simulink model "Comparison_to_Nest_Synapse"  (R2020b)
settings: Solver=FixedStepAuto  StartTime=0.0  StopTime=0.4  FixedStep=0.0001  RelTol=1e-3
undefined symbols (not defined in the file or in its folder): heaviside
libraries: NeuroModelerLibrary x9, simulink x3
settings Model: Creator=Александра  LastModifiedBy=Александра

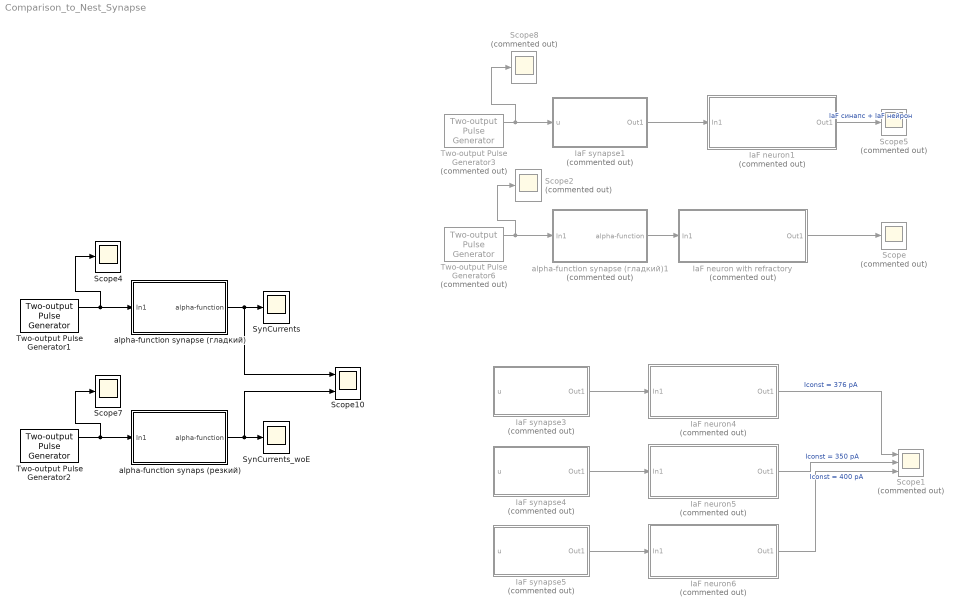
== system Comparison_to_Nest_Synapse ==
  IaF neuron with refractory : Subsystem  Commented=on  mask{tau_m=0.01, Cm=250e-12, I_const=376e-12, E_L=-0.070, V_reset=-0.070, V_th=-0.055, tau_ref=0.002}
      mask prompts: tau_m "Membrane time constatnt"; Cm "Membrane capacity"; I_const "Constant input current"; E_L "Resting membrane potential"; V_reset "Reset membrane potential"; V_th "Threshold potential"; tau_ref "Refractory period"
  IaF neuron1 : Subsystem  Commented=on  mask{tau_m=0.01, Cm=250e-12, I_const=0, E_L=-0.070, V_reset=-0.10, V_th=-0.055}
      mask prompts: tau_m "Membrane time constatnt"; Cm "Membrane capacity"; I_const "Constant input current"; E_L "Resting membrane potential"; V_reset "Reset membrane potential"; V_th "Threshold potential"
  IaF neuron4 : Subsystem  Commented=on  mask{tau_m=0.010, Cm=250e-12, I_const=376e-12, E_L=-0.070, V_reset=-0.070, V_th=-0.055}
      mask prompts: tau_m "Membrane time constatnt"; Cm "Membrane capacity"; I_const "Constant input current"; E_L "Resting membrane potential"; V_reset "Reset membrane potential"; V_th "Threshold potential"
  IaF neuron5 : Subsystem  Commented=on  mask{tau_m=0.010, Cm=250e-12, I_const=350e-12, E_L=-0.070, V_reset=-0.070, V_th=-0.055}
      mask prompts: tau_m "Membrane time constatnt"; Cm "Membrane capacity"; I_const "Constant input current"; E_L "Resting membrane potential"; V_reset "Reset membrane potential"; V_th "Threshold potential"
  IaF neuron6 : Subsystem  Commented=on  mask{tau_m=0.010, Cm=250e-12, I_const=400e-12, E_L=-0.070, V_reset=-0.070, V_th=-0.055}
      mask prompts: tau_m "Membrane time constatnt"; Cm "Membrane capacity"; I_const "Constant input current"; E_L "Resting membrane potential"; V_reset "Reset membrane potential"; V_th "Threshold potential"
  IaF synapse1 : Subsystem  Commented=on  mask{tau_syn=2e-3, I_syn=1, weight=1, delay=1e-3}
      mask prompts: tau_syn "Rise time of the excitatory synaptic alpha function"; I_syn "Synaptic current amplitude"
  IaF synapse3 : Subsystem  Commented=on  mask{tau_syn=2e-3, I_syn=1e-8, weight=1, delay=1e-3}
      mask prompts: tau_syn "Rise time of the excitatory synaptic alpha function"; I_syn "Synaptic current amplitude"
  IaF synapse4 : Subsystem  Commented=on  mask{tau_syn=2e-3, I_syn=1e-8, weight=1, delay=1e-3}
      mask prompts: tau_syn "Rise time of the excitatory synaptic alpha function"; I_syn "Synaptic current amplitude"
  IaF synapse5 : Subsystem  Commented=on  mask{tau_syn=2e-3, I_syn=1e-8, weight=1, delay=1e-3}
      mask prompts: tau_syn "Rise time of the excitatory synaptic alpha function"; I_syn "Synaptic current amplitude"
  Scope{,2,5,8} (4 alike) : Scope  Commented=on
  Scope1 : Scope  Commented=on  NumInputPorts=3
  Scope10 : Scope  NumInputPorts=2
  Scope4 : Scope
  Scope7 : Scope
  SynCurrents : Scope
  SynCurrents_woE : Scope
  Two-output Pulse Generator1 : NeuroModelerLibrary/Support/Two-output Pulse Generator  A=1  P1=200  P2=200  PW=1  ST=0.001  OOn1=0.1  OOff1=1.0  OOn2=0.1  OOff2=0.2
  Two-output Pulse Generator2 : NeuroModelerLibrary/Support/Two-output Pulse Generator  A=1  P1=200  P2=200  PW=1  ST=0.001  OOn1=0.1  OOff1=1.0  OOn2=0.1  OOff2=0.2
  Two-output Pulse Generator3 : NeuroModelerLibrary/Support/Two-output Pulse Generator  Commented=on  A=1  P1=200  P2=200  PW=1  ST=0.001  OOn1=0.1  OOff1=1.0  OOn2=0.1  OOff2=0.2
  Two-output Pulse Generator6 : NeuroModelerLibrary/Support/Two-output Pulse Generator  Commented=on  A=1  P1=200  P2=200  PW=1  ST=0.001  OOn1=0.1  OOff1=1.0  OOn2=0.1  OOff2=0.2
  alpha-function synaps (резкий) : Subsystem
  alpha-function synapse (гладкий) : Subsystem
  alpha-function synapse (гладкий)1 : Subsystem  Commented=on
  wires:
  alpha-function synapse (гладкий)1/1(alpha-function) -> IaF neuron with refractory/1(In1)
  IaF neuron4/1(Out1) -> Scope1/1  "Iconst = 376 pA"
  IaF synapse3/1(Out1) -> IaF neuron4/1(In1)
  IaF synapse4/1(Out1) -> IaF neuron5/1(In1)
  IaF synapse5/1(Out1) -> IaF neuron6/1(In1)
  IaF neuron5/1(Out1) -> Scope1/2  "Iconst = 350 pA"
  IaF neuron6/1(Out1) -> Scope1/3  "Iconst = 400 pA"
  alpha-function synapse (гладкий)/1(alpha-function) -> Scope10/1, SynCurrents/1
  Two-output Pulse Generator1/1 -> Scope4/1, alpha-function synapse (гладкий)/1(In1)
  Two-output Pulse Generator2/1 -> Scope7/1, alpha-function synaps (резкий)/1(In1)
  alpha-function synaps (резкий)/1(alpha-function) -> Scope10/2, SynCurrents_woE/1
  Two-output Pulse Generator6/1 -> alpha-function synapse (гладкий)1/1(In1), Scope2/1
  IaF neuron1/1(Out1) -> Scope5/1  "IaF синапс + IaF нейрон"
  IaF synapse1/1(Out1) -> IaF neuron1/1(In1)
  Two-output Pulse Generator3/1 -> Scope8/1, IaF synapse1/1(u)
  IaF neuron with refractory/1(Out1) -> Scope/1

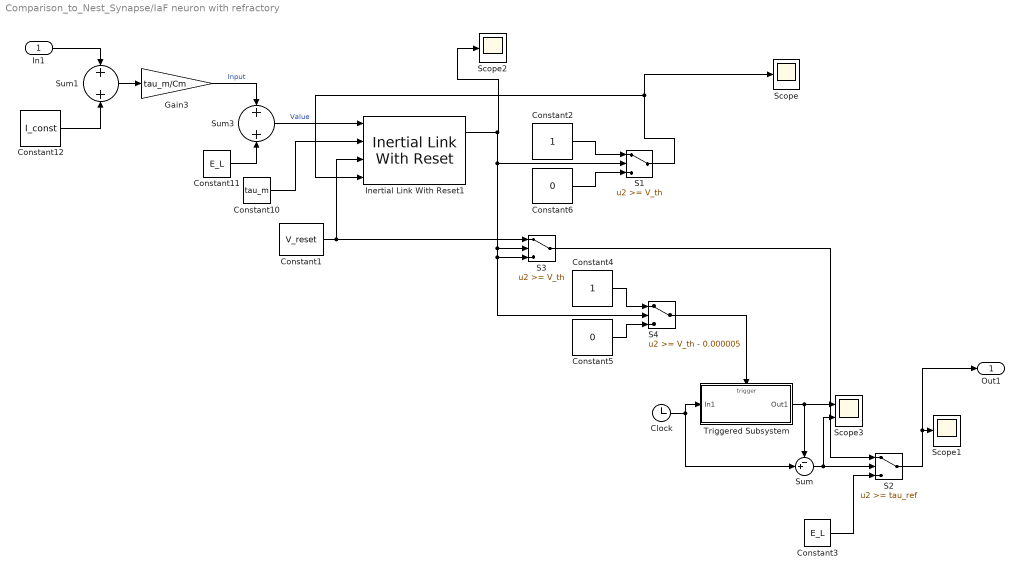
== system Comparison_to_Nest_Synapse/IaF neuron with refractory ==
  In1 : Inport
  Clock : Clock
  Constant1 : Constant  Value=V_reset
  Constant10 : Constant  Value=tau_m
  Constant11 : Constant  Value=E_L
  Constant12 : Constant  Value=I_const
  Constant2 : Constant
  Constant3 : Constant  Value=E_L
  Constant4 : Constant
  Constant5 : Constant  Value=0
  Constant6 : Constant  Value=0
  Gain3 : Gain  Gain=tau_m/Cm
  Inertial Link With Reset1 : NeuroModelerLibrary/Support/Inertial Link With Reset  SystemSampleTime=-1  VariantActivationTime=update diagram  Latency=0  AutoFrameSizeCalculation=off
  S1 : Switch  Threshold=V_th  SaturateOnIntegerOverflow=on  InputSameDT=on
  S2 : Switch  Threshold=tau_ref  SaturateOnIntegerOverflow=on  InputSameDT=on
  S3 : Switch  Threshold=V_th  SaturateOnIntegerOverflow=on  InputSameDT=on
  S4 : Switch  Threshold=V_th - 0.000005  SaturateOnIntegerOverflow=on  InputSameDT=on
  Scope : Scope
  Scope1 : Scope
  Scope2 : Scope
  Scope3 : Scope  NumInputPorts=2
  Sum : Sum  Inputs=-+|
  Sum1 : Sum
  Sum3 : Sum
  Triggered Subsystem : Subsystem  TreatAsAtomicUnit=on
  Out1 : Outport
  wires:
  Constant11/1 -> Sum3/2
  Constant10/1 -> Inertial Link With Reset1/2
  In1/1 -> Sum1/1
  Sum1/1 -> Gain3/1
  Constant12/1 -> Sum1/2
  Constant2/1 -> S1/1
  Constant6/1 -> S1/3
  Sum3/1 -> Inertial Link With Reset1/1  "Value"
  Constant1/1 -> S3/1, Inertial Link With Reset1/3
  S1/1 -> Inertial Link With Reset1/4, Scope/1
  S3/1 -> S2/1
  Gain3/1 -> Sum3/1  "Input"
  Triggered Subsystem/1(Out1) -> Scope3/1, Sum/1
  Clock/1 -> Sum/2, Triggered Subsystem/1(In1)
  Sum/1 -> Scope3/2, S2/2
  S2/1 -> Out1/1, Scope1/1
  Constant3/1 -> S2/3
  Constant4/1 -> S4/1
  Inertial Link With Reset1/1 -> Scope2/1, S4/2, S3/3, S3/2, S1/2
  Constant5/1 -> S4/3
  S4/1 -> Triggered Subsystem/Trigger

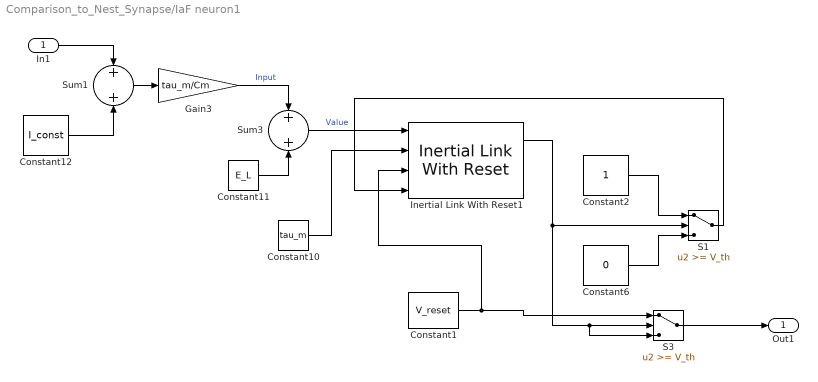
== system Comparison_to_Nest_Synapse/IaF neuron1 ==
  In1 : Inport
  Constant1 : Constant  Value=V_reset
  Constant10 : Constant  Value=tau_m
  Constant11 : Constant  Value=E_L
  Constant12 : Constant  Value=I_const
  Constant2 : Constant
  Constant6 : Constant  Value=0
  Gain3 : Gain  Gain=tau_m/Cm
  Inertial Link With Reset1 : NeuroModelerLibrary/Support/Inertial Link With Reset  SystemSampleTime=-1  VariantActivationTime=update diagram  Latency=0  AutoFrameSizeCalculation=off
  S1 : Switch  Threshold=V_th  SaturateOnIntegerOverflow=on  InputSameDT=on
  S3 : Switch  Threshold=V_th  SaturateOnIntegerOverflow=on  InputSameDT=on
  Sum1 : Sum
  Sum3 : Sum
  Out1 : Outport
  wires:
  Constant11/1 -> Sum3/2
  Constant10/1 -> Inertial Link With Reset1/2
  In1/1 -> Sum1/1
  Sum1/1 -> Gain3/1
  Constant12/1 -> Sum1/2
  Constant2/1 -> S1/1
  Constant6/1 -> S1/3
  Sum3/1 -> Inertial Link With Reset1/1  "Value"
  Inertial Link With Reset1/1 -> S1/2, S3/3, S3/2
  Constant1/1 -> Inertial Link With Reset1/3, S3/1
  S1/1 -> Inertial Link With Reset1/4
  S3/1 -> Out1/1
  Gain3/1 -> Sum3/1  "Input"

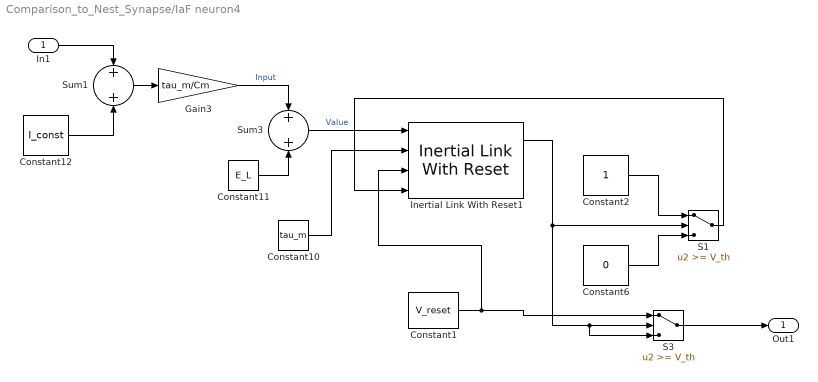
== system Comparison_to_Nest_Synapse/IaF neuron4 ==
  In1 : Inport
  Constant1 : Constant  Value=V_reset
  Constant10 : Constant  Value=tau_m
  Constant11 : Constant  Value=E_L
  Constant12 : Constant  Value=I_const
  Constant2 : Constant
  Constant6 : Constant  Value=0
  Gain3 : Gain  Gain=tau_m/Cm
  Inertial Link With Reset1 : NeuroModelerLibrary/Support/Inertial Link With Reset  SystemSampleTime=-1  VariantActivationTime=update diagram  Latency=0  AutoFrameSizeCalculation=off
  S1 : Switch  Threshold=V_th  SaturateOnIntegerOverflow=on  InputSameDT=on
  S3 : Switch  Threshold=V_th  SaturateOnIntegerOverflow=on  InputSameDT=on
  Sum1 : Sum
  Sum3 : Sum
  Out1 : Outport
  wires:
  Constant11/1 -> Sum3/2
  Constant10/1 -> Inertial Link With Reset1/2
  In1/1 -> Sum1/1
  Sum1/1 -> Gain3/1
  Constant12/1 -> Sum1/2
  Constant2/1 -> S1/1
  Constant6/1 -> S1/3
  Sum3/1 -> Inertial Link With Reset1/1  "Value"
  Inertial Link With Reset1/1 -> S1/2, S3/3, S3/2
  Constant1/1 -> Inertial Link With Reset1/3, S3/1
  S1/1 -> Inertial Link With Reset1/4
  S3/1 -> Out1/1
  Gain3/1 -> Sum3/1  "Input"

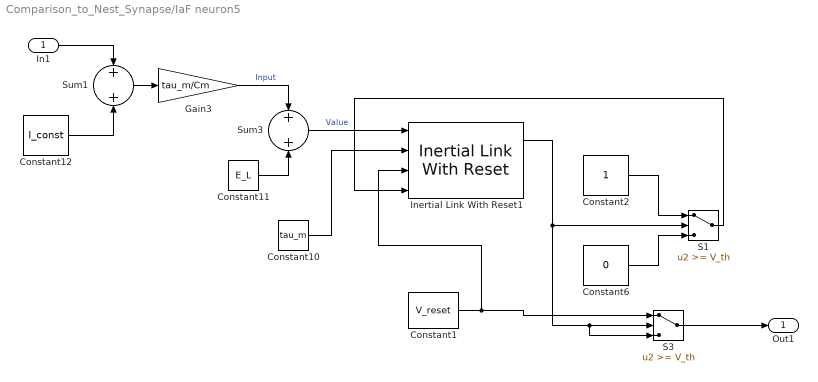
== system Comparison_to_Nest_Synapse/IaF neuron5 ==
  In1 : Inport
  Constant1 : Constant  Value=V_reset
  Constant10 : Constant  Value=tau_m
  Constant11 : Constant  Value=E_L
  Constant12 : Constant  Value=I_const
  Constant2 : Constant
  Constant6 : Constant  Value=0
  Gain3 : Gain  Gain=tau_m/Cm
  Inertial Link With Reset1 : NeuroModelerLibrary/Support/Inertial Link With Reset  SystemSampleTime=-1  VariantActivationTime=update diagram  Latency=0  AutoFrameSizeCalculation=off
  S1 : Switch  Threshold=V_th  SaturateOnIntegerOverflow=on  InputSameDT=on
  S3 : Switch  Threshold=V_th  SaturateOnIntegerOverflow=on  InputSameDT=on
  Sum1 : Sum
  Sum3 : Sum
  Out1 : Outport
  wires:
  Constant11/1 -> Sum3/2
  Constant10/1 -> Inertial Link With Reset1/2
  In1/1 -> Sum1/1
  Sum1/1 -> Gain3/1
  Constant12/1 -> Sum1/2
  Constant2/1 -> S1/1
  Constant6/1 -> S1/3
  Sum3/1 -> Inertial Link With Reset1/1  "Value"
  Inertial Link With Reset1/1 -> S1/2, S3/3, S3/2
  Constant1/1 -> Inertial Link With Reset1/3, S3/1
  S1/1 -> Inertial Link With Reset1/4
  S3/1 -> Out1/1
  Gain3/1 -> Sum3/1  "Input"

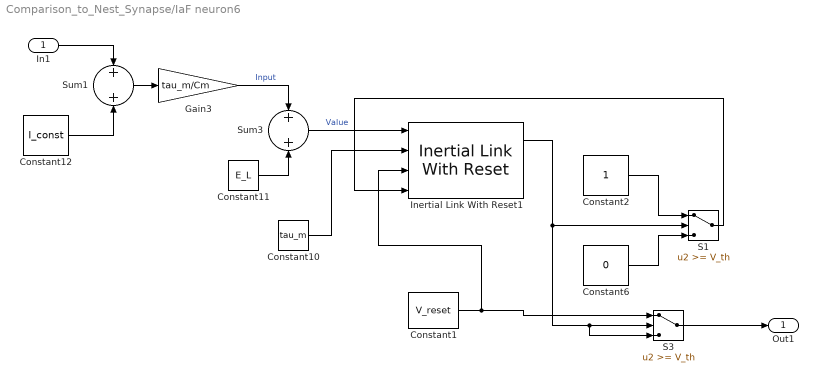
== system Comparison_to_Nest_Synapse/IaF neuron6 ==
  In1 : Inport
  Constant1 : Constant  Value=V_reset
  Constant10 : Constant  Value=tau_m
  Constant11 : Constant  Value=E_L
  Constant12 : Constant  Value=I_const
  Constant2 : Constant
  Constant6 : Constant  Value=0
  Gain3 : Gain  Gain=tau_m/Cm
  Inertial Link With Reset1 : NeuroModelerLibrary/Support/Inertial Link With Reset  SystemSampleTime=-1  VariantActivationTime=update diagram  Latency=0  AutoFrameSizeCalculation=off
  S1 : Switch  Threshold=V_th  SaturateOnIntegerOverflow=on  InputSameDT=on
  S3 : Switch  Threshold=V_th  SaturateOnIntegerOverflow=on  InputSameDT=on
  Sum1 : Sum
  Sum3 : Sum
  Out1 : Outport
  wires:
  Constant11/1 -> Sum3/2
  Constant10/1 -> Inertial Link With Reset1/2
  In1/1 -> Sum1/1
  Sum1/1 -> Gain3/1
  Constant12/1 -> Sum1/2
  Constant2/1 -> S1/1
  Constant6/1 -> S1/3
  Sum3/1 -> Inertial Link With Reset1/1  "Value"
  Inertial Link With Reset1/1 -> S1/2, S3/3, S3/2
  Constant1/1 -> Inertial Link With Reset1/3, S3/1
  S1/1 -> Inertial Link With Reset1/4
  S3/1 -> Out1/1
  Gain3/1 -> Sum3/1  "Input"

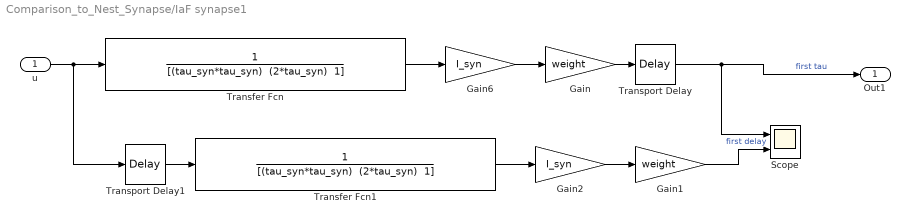
== system Comparison_to_Nest_Synapse/IaF synapse1 ==
  u : Inport
  Gain : Gain  Gain=weight
  Gain1 : Gain  Gain=weight
  Gain2 : Gain  Gain=I_syn
  Gain6 : Gain  Gain=I_syn
  Scope : Scope  NumInputPorts=2
  Transfer Fcn : TransferFcn  Denominator="[(tau_syn*tau_syn)  (2*tau_syn)  1]"
  Transfer Fcn1 : TransferFcn  Denominator="[(tau_syn*tau_syn)  (2*tau_syn)  1]"
  Transport Delay : TransportDelay  DelayTime=delay
  Transport Delay1 : TransportDelay  DelayTime=delay
  Out1 : Outport
  wires:
  Transport Delay/1 -> Scope/1, Out1/1  "first tau"
  Gain/1 -> Transport Delay/1
  Gain6/1 -> Gain/1
  Transfer Fcn/1 -> Gain6/1
  u/1 -> Transport Delay1/1, Transfer Fcn/1
  Transfer Fcn1/1 -> Gain2/1
  Gain2/1 -> Gain1/1
  Transport Delay1/1 -> Transfer Fcn1/1
  Gain1/1 -> Scope/2  "first delay"

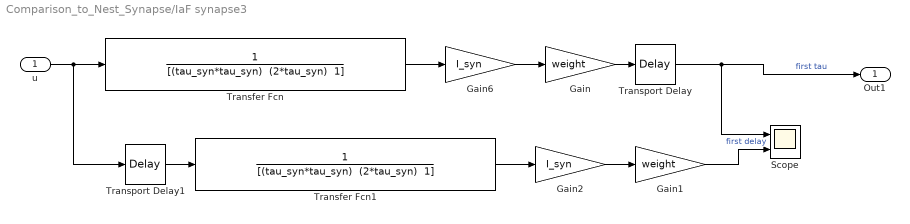
== system Comparison_to_Nest_Synapse/IaF synapse3 ==
  u : Inport
  Gain : Gain  Gain=weight
  Gain1 : Gain  Gain=weight
  Gain2 : Gain  Gain=I_syn
  Gain6 : Gain  Gain=I_syn
  Scope : Scope  NumInputPorts=2
  Transfer Fcn : TransferFcn  Denominator="[(tau_syn*tau_syn)  (2*tau_syn)  1]"
  Transfer Fcn1 : TransferFcn  Denominator="[(tau_syn*tau_syn)  (2*tau_syn)  1]"
  Transport Delay : TransportDelay  DelayTime=delay
  Transport Delay1 : TransportDelay  DelayTime=delay
  Out1 : Outport
  wires:
  Transport Delay/1 -> Scope/1, Out1/1  "first tau"
  Gain/1 -> Transport Delay/1
  Gain6/1 -> Gain/1
  Transfer Fcn/1 -> Gain6/1
  u/1 -> Transport Delay1/1, Transfer Fcn/1
  Transfer Fcn1/1 -> Gain2/1
  Gain2/1 -> Gain1/1
  Transport Delay1/1 -> Transfer Fcn1/1
  Gain1/1 -> Scope/2  "first delay"

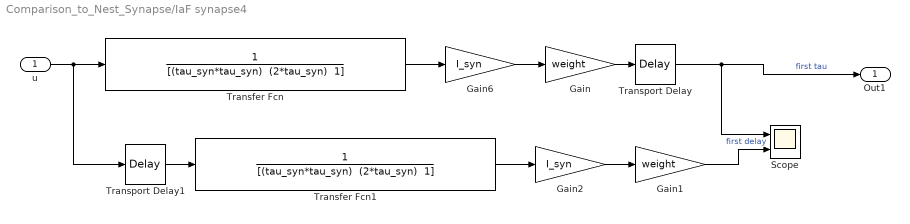
== system Comparison_to_Nest_Synapse/IaF synapse4 ==
  u : Inport
  Gain : Gain  Gain=weight
  Gain1 : Gain  Gain=weight
  Gain2 : Gain  Gain=I_syn
  Gain6 : Gain  Gain=I_syn
  Scope : Scope  NumInputPorts=2
  Transfer Fcn : TransferFcn  Denominator="[(tau_syn*tau_syn)  (2*tau_syn)  1]"
  Transfer Fcn1 : TransferFcn  Denominator="[(tau_syn*tau_syn)  (2*tau_syn)  1]"
  Transport Delay : TransportDelay  DelayTime=delay
  Transport Delay1 : TransportDelay  DelayTime=delay
  Out1 : Outport
  wires:
  Transport Delay/1 -> Scope/1, Out1/1  "first tau"
  Gain/1 -> Transport Delay/1
  Gain6/1 -> Gain/1
  Transfer Fcn/1 -> Gain6/1
  u/1 -> Transport Delay1/1, Transfer Fcn/1
  Transfer Fcn1/1 -> Gain2/1
  Gain2/1 -> Gain1/1
  Transport Delay1/1 -> Transfer Fcn1/1
  Gain1/1 -> Scope/2  "first delay"

== system Comparison_to_Nest_Synapse/IaF synapse5 ==
  u : Inport
  Gain : Gain  Gain=weight
  Gain1 : Gain  Gain=weight
  Gain2 : Gain  Gain=I_syn
  Gain6 : Gain  Gain=I_syn
  Scope : Scope  NumInputPorts=2
  Transfer Fcn : TransferFcn  Denominator="[(tau_syn*tau_syn)  (2*tau_syn)  1]"
  Transfer Fcn1 : TransferFcn  Denominator="[(tau_syn*tau_syn)  (2*tau_syn)  1]"
  Transport Delay : TransportDelay  DelayTime=delay
  Transport Delay1 : TransportDelay  DelayTime=delay
  Out1 : Outport
  wires:
  Transport Delay/1 -> Scope/1, Out1/1  "first tau"
  Gain/1 -> Transport Delay/1
  Gain6/1 -> Gain/1
  Transfer Fcn/1 -> Gain6/1
  u/1 -> Transport Delay1/1, Transfer Fcn/1
  Transfer Fcn1/1 -> Gain2/1
  Gain2/1 -> Gain1/1
  Transport Delay1/1 -> Transfer Fcn1/1
  Gain1/1 -> Scope/2  "first delay"

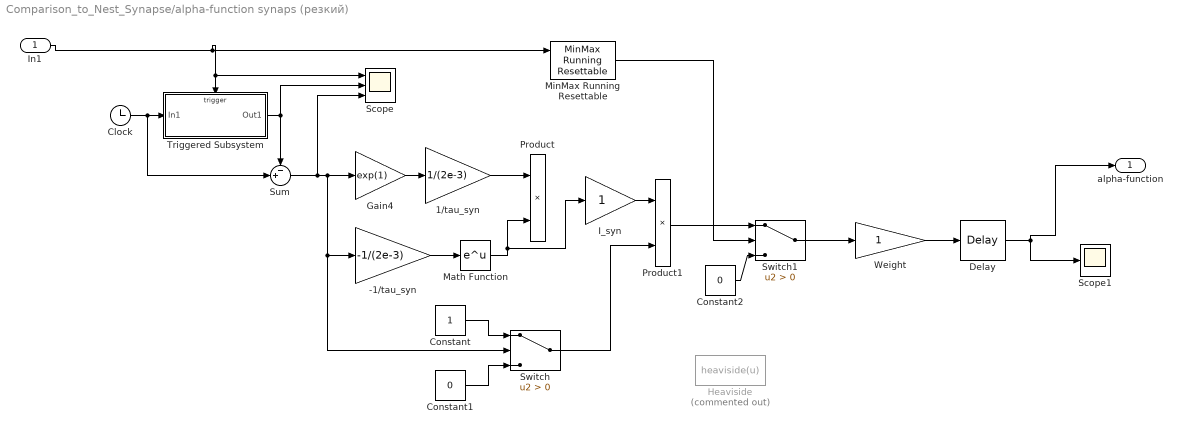
== system Comparison_to_Nest_Synapse/alpha-function synaps (резкий) ==
  In1 : Inport
  -1/tau_syn : Gain  Gain=-1/(2e-3)
  1/tau_syn : Gain  Gain=1/(2e-3)
  Clock : Clock
  Constant : Constant
  Constant1 : Constant  Value=0
  Constant2 : Constant  Value=0
  Delay : TransportDelay  DelayTime=0.001
  Gain4 : Gain  Gain=exp(1)
  Heaviside : MATLABFcn  Commented=on  MATLABFcn=heaviside(u)  OutputSignalType=real  Output1D=off
  I_syn : Gain
  Math Function : Math  SaturateOnIntegerOverflow=on
  MinMax Running Resettable : simulink/Math Operations/MinMax Running Resettable  Function=max  vinit=0.0
  Product : Product
  Product1 : Product
  Scope : Scope  NumInputPorts=3
  Scope1 : Scope
  Sum : Sum  Inputs=-+|
  Switch : Switch  Criteria=u2 > Threshold
  Switch1 : Switch  Criteria=u2 > Threshold
  Triggered Subsystem : Subsystem  TreatAsAtomicUnit=on
  Weight : Gain
  alpha-function : Outport
  wires:
  I_syn/1 -> Product1/1
  1/tau_syn/1 -> Product/1
  Weight/1 -> Delay/1
  Sum/1 -> Scope/3, Switch/2, -1/tau_syn/1, Gain4/1
  Gain4/1 -> 1/tau_syn/1
  -1/tau_syn/1 -> Math Function/1
  Math Function/1 -> I_syn/1, Product/2
  Switch/1 -> Product1/2
  Clock/1 -> Sum/2, Triggered Subsystem/1(In1)
  In1/1 -> Scope/1, Triggered Subsystem/Trigger, MinMax Running Resettable/1
  Triggered Subsystem/1(Out1) -> Sum/1, Scope/2
  Constant1/1 -> Switch/3
  Constant/1 -> Switch/1
  Constant2/1 -> Switch1/3
  Product1/1 -> Switch1/1
  MinMax Running Resettable/1 -> Switch1/2
  Switch1/1 -> Weight/1
  Delay/1 -> alpha-function/1, Scope1/1

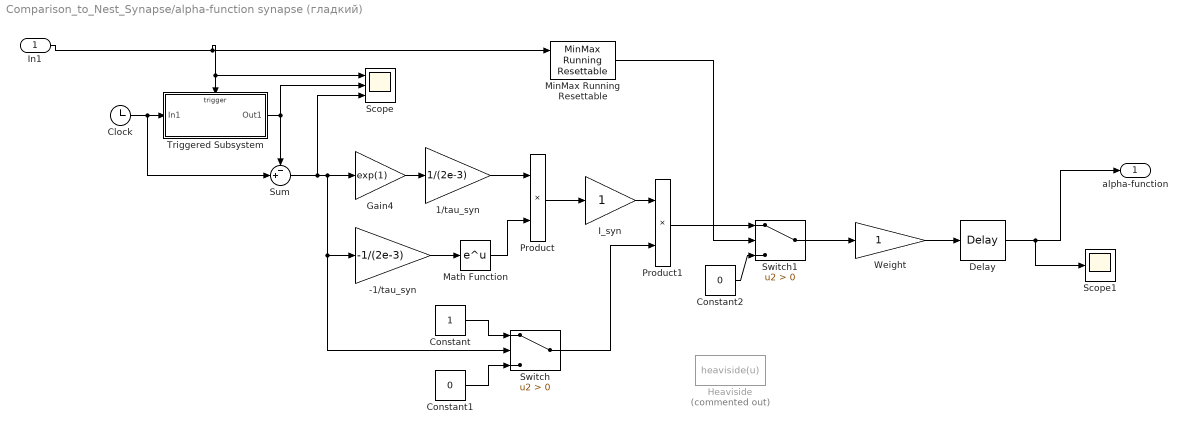
== system Comparison_to_Nest_Synapse/alpha-function synapse (гладкий) ==
  In1 : Inport
  -1/tau_syn : Gain  Gain=-1/(2e-3)
  1/tau_syn : Gain  Gain=1/(2e-3)
  Clock : Clock
  Constant : Constant
  Constant1 : Constant  Value=0
  Constant2 : Constant  Value=0
  Delay : TransportDelay  DelayTime=0.001
  Gain4 : Gain  Gain=exp(1)
  Heaviside : MATLABFcn  Commented=on  MATLABFcn=heaviside(u)  OutputSignalType=real  Output1D=off
  I_syn : Gain
  Math Function : Math  SaturateOnIntegerOverflow=on
  MinMax Running Resettable : simulink/Math Operations/MinMax Running Resettable  Function=max  vinit=0.0
  Product : Product
  Product1 : Product
  Scope : Scope  NumInputPorts=3
  Scope1 : Scope
  Sum : Sum  Inputs=-+|
  Switch : Switch  Criteria=u2 > Threshold
  Switch1 : Switch  Criteria=u2 > Threshold
  Triggered Subsystem : Subsystem  TreatAsAtomicUnit=on
  Weight : Gain
  alpha-function : Outport
  wires:
  I_syn/1 -> Product1/1
  1/tau_syn/1 -> Product/1
  Weight/1 -> Delay/1
  Sum/1 -> Scope/3, Switch/2, -1/tau_syn/1, Gain4/1
  Gain4/1 -> 1/tau_syn/1
  -1/tau_syn/1 -> Math Function/1
  Math Function/1 -> Product/2
  Switch/1 -> Product1/2
  Clock/1 -> Sum/2, Triggered Subsystem/1(In1)
  In1/1 -> Scope/1, Triggered Subsystem/Trigger, MinMax Running Resettable/1
  Triggered Subsystem/1(Out1) -> Sum/1, Scope/2
  Constant1/1 -> Switch/3
  Constant/1 -> Switch/1
  Product/1 -> I_syn/1
  Constant2/1 -> Switch1/3
  Product1/1 -> Switch1/1
  MinMax Running Resettable/1 -> Switch1/2
  Switch1/1 -> Weight/1
  Delay/1 -> Scope1/1, alpha-function/1

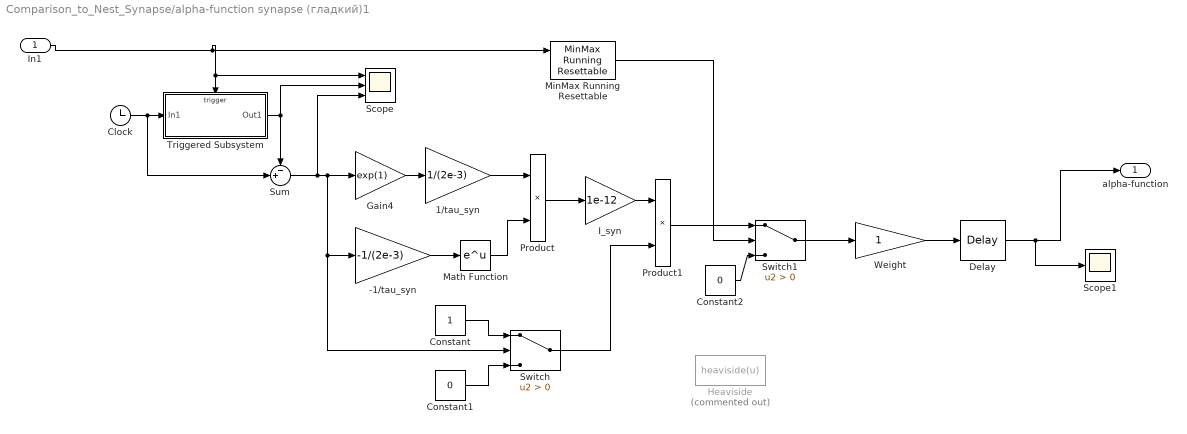
== system Comparison_to_Nest_Synapse/alpha-function synapse (гладкий)1 ==
  In1 : Inport
  -1/tau_syn : Gain  Gain=-1/(2e-3)
  1/tau_syn : Gain  Gain=1/(2e-3)
  Clock : Clock
  Constant : Constant
  Constant1 : Constant  Value=0
  Constant2 : Constant  Value=0
  Delay : TransportDelay  DelayTime=0.001
  Gain4 : Gain  Gain=exp(1)
  Heaviside : MATLABFcn  Commented=on  MATLABFcn=heaviside(u)  OutputSignalType=real  Output1D=off
  I_syn : Gain  Gain=1e-12
  Math Function : Math  SaturateOnIntegerOverflow=on
  MinMax Running Resettable : simulink/Math Operations/MinMax Running Resettable  Function=max  vinit=0.0
  Product : Product
  Product1 : Product
  Scope : Scope  NumInputPorts=3
  Scope1 : Scope
  Sum : Sum  Inputs=-+|
  Switch : Switch  Criteria=u2 > Threshold
  Switch1 : Switch  Criteria=u2 > Threshold
  Triggered Subsystem : Subsystem  TreatAsAtomicUnit=on
  Weight : Gain
  alpha-function : Outport
  wires:
  I_syn/1 -> Product1/1
  1/tau_syn/1 -> Product/1
  Weight/1 -> Delay/1
  Sum/1 -> Scope/3, Switch/2, -1/tau_syn/1, Gain4/1
  Gain4/1 -> 1/tau_syn/1
  -1/tau_syn/1 -> Math Function/1
  Math Function/1 -> Product/2
  Switch/1 -> Product1/2
  Clock/1 -> Sum/2, Triggered Subsystem/1(In1)
  In1/1 -> Scope/1, Triggered Subsystem/Trigger, MinMax Running Resettable/1
  Triggered Subsystem/1(Out1) -> Sum/1, Scope/2
  Constant1/1 -> Switch/3
  Constant/1 -> Switch/1
  Product/1 -> I_syn/1
  Constant2/1 -> Switch1/3
  Product1/1 -> Switch1/1
  MinMax Running Resettable/1 -> Switch1/2
  Switch1/1 -> Weight/1
  Delay/1 -> Scope1/1, alpha-function/1

== system Comparison_to_Nest_Synapse/IaF neuron with refractory/Triggered Subsystem ==
  In1 : Inport
  Trigger : TriggerPort  VariantControl=Variant
  Out1 : Outport
  wires:
  In1/1 -> Out1/1

== system Comparison_to_Nest_Synapse/alpha-function synaps (резкий)/Triggered Subsystem ==
  In1 : Inport
  Trigger : TriggerPort  VariantControl=Variant
  Out1 : Outport
  wires:
  In1/1 -> Out1/1

== system Comparison_to_Nest_Synapse/alpha-function synapse (гладкий)/Triggered Subsystem ==
  In1 : Inport
  Trigger : TriggerPort  VariantControl=Variant
  Out1 : Outport
  wires:
  In1/1 -> Out1/1

== system Comparison_to_Nest_Synapse/alpha-function synapse (гладкий)1/Triggered Subsystem ==
  In1 : Inport
  Trigger : TriggerPort  VariantControl=Variant
  Out1 : Outport
  wires:
  In1/1 -> Out1/1
